simulink model "Dc_mot"  (R2019b)
settings: Solver=VariableStepAuto  StartTime=0.0  StopTime=1  MaxStep=1e-6  RelTol=1e-6
InitFcn:
  | Ra = 1.2; % Armature resistance
  | La = 2.5e-3; %armature inductance
  | Kc = 0.35; %flux constant
  | J = 1e-3; % moment of inertia
  | %% Gains of the 2DOF PI current controller
  | alphac = 2*pi*500; %closed loop bandwidth
  | Kpc = alphac*La; % proportional gain
  | Kic = alphac*2*La; %integral gain
  | r = Kpc- Ra; %active resistance
  | Umax = 72; %saturation: upper limit
  | Umin = -72; %saturation lower limit
libraries: simulink x2
settings Model: Creator=srikesh  LastModifiedBy=srikesh

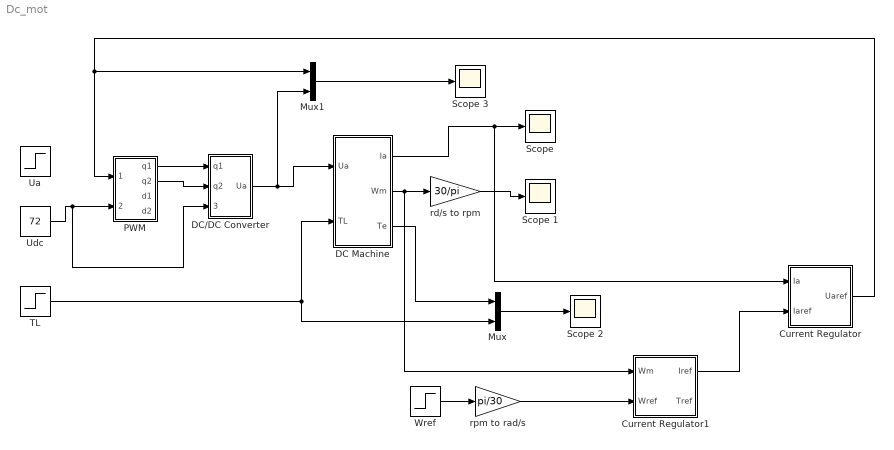
== system Dc_mot ==
  Current Regulator : Subsystem
  Current Regulator1 : Subsystem
  "DC Machine " : Subsystem  mask{Ra=1.2, La=2.5e-3, J=1e-3, fr=5e-2, Ke=.35, Kc=.35}
      mask prompts: Ra "Ra(Ohm)"; La "La(H)"; J "J(N-ms^-1)"; fr "fr(N.ms)"; Ke "Ke(V.s)"; Kc "Kc(NmA^1)"
  DC/DC Converter : Subsystem
  Mux : Mux  Inputs=2
  Mux1 : Mux  Inputs=2
  "PWM " : Subsystem
  Scope {,1..3} (4 alike) : Scope
  TL : Step  Time=.5  After=7  SampleTime=0
  "Ua " : Step  Time=.1  After=120  SampleTime=0
  "Udc " : Constant  Value=72
  Wref : Step  Time=.1  After=2000  SampleTime=0
  "rd/s to rpm " : Gain  Gain=30/pi
  rpm to rad/s : Gain  Gain=pi/30
  wires:
  "DC Machine "/1(Ia) -> Current Regulator/1(Ia), "Scope "/1
  "DC Machine "/2("Wm ") -> Current Regulator1/1(Wm), "rd/s to rpm "/1
  "rd/s to rpm "/1 -> Scope 1/1
  "PWM "/1(q1) -> DC/DC Converter/1("q1 ")
  "PWM "/2(q2) -> DC/DC Converter/2("q2 ")
  TL/1 -> "DC Machine "/2("TL "), Mux/2
  "Udc "/1 -> DC/DC Converter/3("Udc "), "PWM "/2("Udc ")
  "DC Machine "/3("Te ") -> Mux/1
  Mux/1 -> Scope 2/1
  DC/DC Converter/1("Ua ") -> Mux1/2, "DC Machine "/1("Ua ")
  Mux1/1 -> Scope 3/1
  Wref/1 -> rpm to rad/s/1
  rpm to rad/s/1 -> Current Regulator1/2("Wref ")
  Current Regulator1/1("Iref ") -> Current Regulator/2("Iaref ")
  Current Regulator/1(" Uaref ") -> "PWM "/1("Uaref "), Mux1/1

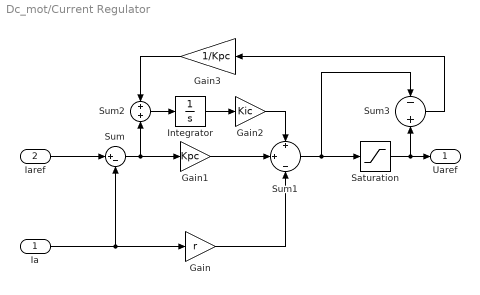
== system Dc_mot/Current Regulator ==
  Ia : Inport
  "Iaref " : Inport  Port=2
  Gain : Gain  Gain=r
  Gain1 : Gain  Gain=Kpc
  Gain2 : Gain  Gain=Kic
  Gain3 : Gain  Gain=1/Kpc
  Integrator : Integrator
  Saturation : Saturate  UpperLimit=Umax  LowerLimit=-Umin
  Sum : Sum  Inputs=|+-
  Sum1 : Sum  Inputs=+|+|-
  Sum2 : Sum  Inputs=+|+
  Sum3 : Sum  Inputs=-|+
  " Uaref " : Outport
  wires:
  "Iaref "/1 -> Sum/1
  Ia/1 -> Gain/1, Sum/2
  Sum/1 -> Sum2/2, Gain1/1
  Integrator/1 -> Gain2/1
  Sum2/1 -> Integrator/1
  Gain3/1 -> Sum2/1
  Gain1/1 -> Sum1/2
  Gain/1 -> Sum1/3
  Gain2/1 -> Sum1/1
  Sum1/1 -> Sum3/1, Saturation/1
  Saturation/1 -> Sum3/2, " Uaref "/1
  Sum3/1 -> Gain3/1

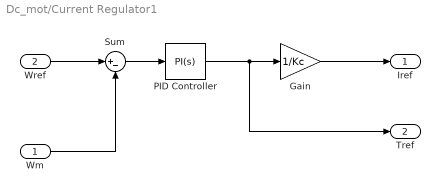
== system Dc_mot/Current Regulator1 ==
  Wm : Inport
  "Wref " : Inport  Port=2
  Gain : Gain  Gain=1/Kc
  PID Controller : simulink/Continuous/PID Controller  Controller=PI  Form=Parallel  TimeDomain=Continuous-time  SampleTime=-1  IntegratorMethod=Forward Euler  FilterMethod=Forward Euler  ControllerParametersSource=internal  P=5  I=0.1  D=0  UseFilter=on  N=100  TunerSelectOption=Transfer Function Based (PID Tuner App)  InitialConditionSource=internal  InitialConditionForIntegrator=0  InitialConditionForFilter=0  DifferentiatorICPrevScaledInput=0  ExternalReset=none  TrackingMode=off  Kt=1  LimitOutput=off  UpperSaturationLimit=inf  LowerSaturationLimit=-inf  LinearizeAsGain=on  AntiWindupMode=none  Kb=1  POutMin=[]  POutMax=[]  IOutMin=[]  IOutMax=[]  DOutMin=[]  DOutMax=[]  NOutMin=[]  NOutMax=[]  SumOutMin=[]  SumOutMax=[]  SaturationOutMin=[]  SaturationOutMax=[]  PParamMin=[]  PParamMax=[]  IParamMin=[]  IParamMax=[]  DParamMin=[]  DParamMax=[]  NParamMin=[]  NParamMax=[]  KbParamMin=[]  KbParamMax=[]  KtParamMin=[]  KtParamMax=[]  KbOutMin=[]  KbOutMax=[]  KtOutMin=[]  KtOutMax=[]  IntegratorOutMin=[]  IntegratorOutMax=[]  FilterOutMin=[]  FilterOutMax=[]  SumI1OutMin=[]  SumI1OutMax=[]  SumI2OutMin=[]  SumI2OutMax=[]  SumI3OutMin=[]  SumI3OutMax=[]  SumI4OutMin=[]  SumI4OutMax=[]  SumDOutMin=[]  SumDOutMax=[]  DifferentiatorOutMin=[]  DifferentiatorOutMax=[]  FilterDiffOutCoefMin=[]  FilterDiffOutCoefMax=[]  ReciprocalOutMin=[]  ReciprocalOutMax=[]  SumDenOutMin=[]  SumDenOutMax=[]  SumNumOutMin=[]  SumNumOutMax=[]  DivideOutMin=[]  DivideOutMax=[]  IntegratorContinuousStateAttributes=''  IntegratorStateMustResolveToSignalObject=off  IntegratorRTWStateStorageClass=Auto  FilterContinuousStateAttributes=''  FilterStateMustResolveToSignalObject=off  FilterRTWStateStorageClass=Auto  ParallelPVariant=InternalParameters  IdealPVariant=Disabled  IVariant=InternalParameters  DVariant=Disabled  IntegratorVariant=Continuous  SatVariant=Disabled  AWVariant=Passthrough  PCopyVariant=Disabled  TRVariant=Disabled  FdbkBlocksVariant=Forward  IdealPFdbkVariant=Disabled  SatFdbkVariant=Disabled  DerivativeFilterVariant=Disabled  NVariant=Disabled  NCopyVariant=Disabled_SignalSpec  FilterICVariant=Disabled  IntegratorICVariant=InternalICs  ExternalResetVariant=Disabled  TRSumVariant=Passthrough  SumFdbkVariant=Disabled  SumVariant=Sum_PI
  Sum : Sum  Inputs=|+-
  "Iref " : Outport
  Tref : Outport  Port=2
  wires:
  "Wref "/1 -> Sum/1
  Wm/1 -> Sum/2
  Sum/1 -> PID Controller/1
  PID Controller/1 -> Tref/1, Gain/1
  Gain/1 -> "Iref "/1

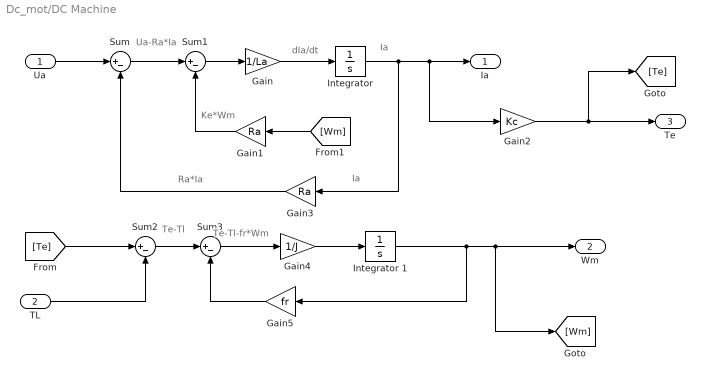
== system Dc_mot/DC Machine  ==
  note: Te-Tl-fr*Wm
  note: Te-Tl
  note: Ke*Wm
  note: Ia
  note: Ra*Ia
  note: Ua-Ra*Ia
  note: dIa/dt
  note: Ia
  "Ua " : Inport
  "TL " : Inport  Port=2
  Gain : Gain  Gain=1/La
  Gain1 : Gain  Gain=Ra
  Gain2 : Gain  Gain=Kc
  Gain3 : Gain  Gain=Ra
  Gain4 : Gain  Gain=1/J
  Gain5 : Gain  Gain=fr
  "Integrator " : Integrator
  Integrator 1 : Integrator
  Sum{,1..3} (4 alike) : Sum  Inputs=|+-
  Ia : Outport
  "Wm " : Outport  Port=2
  "Te " : Outport  Port=3
  wires:
  Sum3/1 -> Gain4/1
  Sum2/1 -> Sum3/1
  [Te] -> Sum2/1
  Gain4/1 -> Integrator 1/1
  Gain5/1 -> Sum3/2
  Gain3/1 -> Sum/2
  Gain2/1 -> "Te "/1, [Te]
  Integrator 1/1 -> Gain5/1, "Wm "/1, [Wm]
  "TL "/1 -> Sum2/2
  Sum1/1 -> Gain/1
  Sum/1 -> Sum1/1
  [Wm] -> Gain1/1
  "Integrator "/1 -> Gain3/1, Ia/1, Gain2/1
  Gain1/1 -> Sum1/2
  "Ua "/1 -> Sum/1
  Gain/1 -> "Integrator "/1

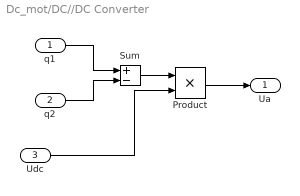
== system Dc_mot/DC//DC Converter ==
  "q1 " : Inport
  "q2 " : Inport  Port=2
  "Udc " : Inport  Port=3
  Product : Product
  Sum : Sum  Inputs=+-
  "Ua " : Outport
  wires:
  "q1 "/1 -> Sum/1
  "q2 "/1 -> Sum/2
  Sum/1 -> Product/1
  "Udc "/1 -> Product/2
  Product/1 -> "Ua "/1

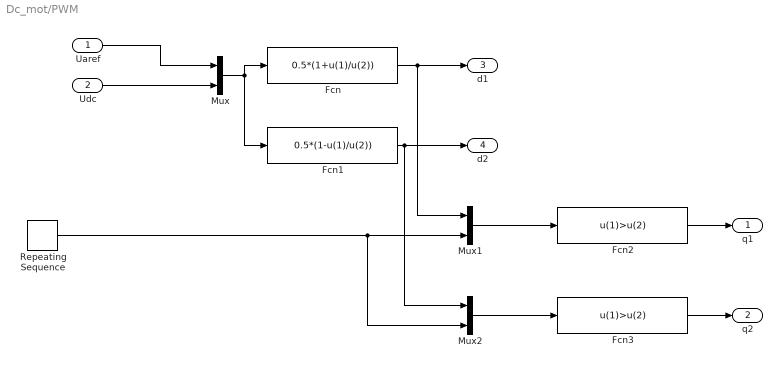
== system Dc_mot/PWM  ==
  "Uaref " : Inport
  "Udc " : Inport  Port=2
  Fcn : Fcn  Expr=0.5*(1+u(1)/u(2))
  Fcn1 : Fcn  Expr=0.5*(1-u(1)/u(2))
  Fcn2 : Fcn  Expr=u(1)>u(2)
  Fcn3 : Fcn  Expr=u(1)>u(2)
  Mux : Mux  Inputs=2
  Mux1 : Mux  Inputs=2
  Mux2 : Mux  Inputs=2
  Repeating Sequence : simulink/Sources/Repeating Sequence  rep_seq_t=[0 100e-6 200e-6]  rep_seq_y=[1 0 1]
  q1 : Outport
  q2 : Outport  Port=2
  "d1 " : Outport  Port=3
  "d2 " : Outport  Port=4
  wires:
  "Uaref "/1 -> Mux/1
  "Udc "/1 -> Mux/2
  Mux/1 -> Fcn1/1, Fcn/1
  Fcn/1 -> Mux1/1, "d1 "/1
  Fcn1/1 -> Mux2/1, "d2 "/1
  Repeating Sequence/1 -> Mux2/2, Mux1/2
  Mux1/1 -> Fcn2/1
  Mux2/1 -> Fcn3/1
  Fcn2/1 -> q1/1
  Fcn3/1 -> q2/1
